simulink model "delta_w_plus"  (Simulink 7.8)
settings: Solver=ode45  StartTime=0.0  StopTime=10.0  RelTol=1e-3
settings Model: Creator=Leo  LastModifiedBy=Leo

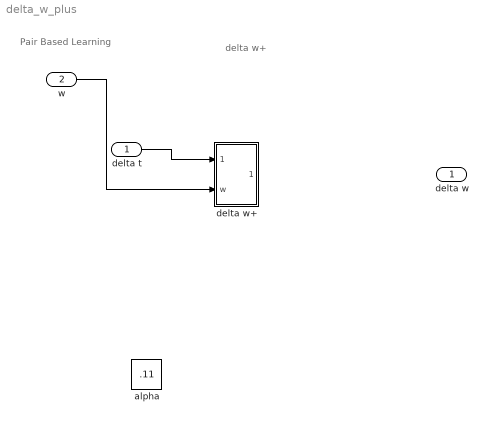
== system delta_w_plus ==
  note: Pair Based Learning
  note: delta w+
  delta t : Inport
  w : Inport  Port=2
  alpha : Constant  Value=.11
  delta w+ : Subsystem
  delta w : Outport
  wires:
  delta t/1 -> delta w+/1(delta t)
  w/1 -> delta w+/2(w)
  ? -> delta w/1

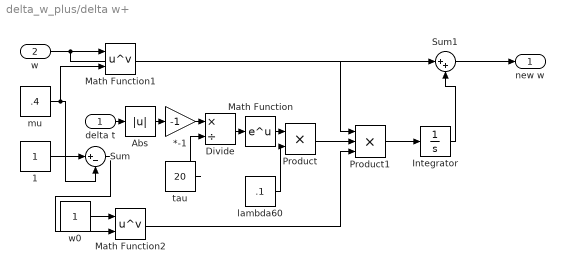
== system delta_w_plus/delta w+ ==
  delta t : Inport
  w : Inport  Port=2
  *-1 : Gain  Gain=-1
  1 : Constant
  Abs : Abs
  Divide : Product  Inputs=*/
  Integrator : Integrator
  Math Function : Math  SaturateOnIntegerOverflow=on
  Math Function1 : Math  Operator=pow  SaturateOnIntegerOverflow=on
  Math Function2 : Math  Operator=pow  SaturateOnIntegerOverflow=on
  Product : Product  Inputs=**
  Product1 : Product  Inputs=***
  Sum : Sum  Inputs=|+-
  Sum1 : Sum  Inputs=|++
  lambda60 : Constant  Value=.1
  mu : Constant  Value=.4
  tau : Constant  Value=20
  w0 : Constant
  new w : Outport
  wires:
  delta t/1 -> Abs/1
  Abs/1 -> *-1/1
  *-1/1 -> Divide/1
  tau/1 -> Divide/2
  Divide/1 -> Math Function/1
  Math Function/1 -> Product/1
  lambda60/1 -> Product/2
  w0/1 -> Math Function2/1
  1/1 -> Sum/1
  mu/1 -> Sum/2, Math Function1/2
  Sum/1 -> Math Function2/2
  w/1 -> Math Function1/1, Sum1/1
  Math Function1/1 -> Product1/1
  Product/1 -> Product1/2
  Math Function2/1 -> Product1/3
  Product1/1 -> Integrator/1
  Integrator/1 -> Sum1/2
  Sum1/1 -> new w/1
